simulink model "modelo_cinematico_inverso"  (R2015a)
settings: Solver=ode45  StartTime=0.0  StopTime=10.0  RelTol=1e-3
settings Model: Creator=samir  LastModifiedBy=samir

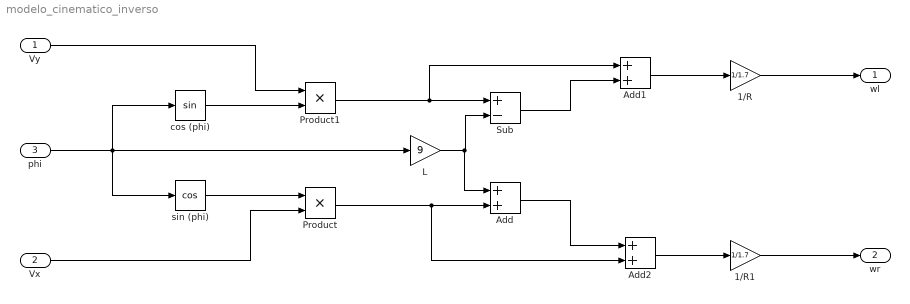
== system modelo_cinematico_inverso ==
  Vy : Inport
  Vx : Inport  Port=2
  phi : Inport  Port=3
  "1/R " : Gain  Gain=1/1.7
  1/R1 : Gain  Gain=1/1.7
  "Add " : Sum
  Add1 : Sum
  Add2 : Sum
  L : Gain  Gain=9
  Product : Product
  Product1 : Product
  Sub : Sum  Inputs=+-
  cos (phi) : Trigonometry
  sin (phi) : Trigonometry  Operator=cos
  wl : Outport
  wr : Outport  Port=2
  wires:
  phi/1 -> sin (phi)/1, L/1, cos (phi)/1
  cos (phi)/1 -> Product1/2
  Vy/1 -> Product1/1
  sin (phi)/1 -> Product/1
  Vx/1 -> Product/2
  Product1/1 -> Add1/1, Sub/1
  L/1 -> "Add "/1, Sub/2
  Product/1 -> Add2/2, "Add "/2
  Sub/1 -> Add1/2
  "Add "/1 -> Add2/1
  Add1/1 -> "1/R "/1
  Add2/1 -> 1/R1/1
  1/R1/1 -> wr/1
  "1/R "/1 -> wl/1
